simulink model "Nonlinear_Inverted_Pendulum_Modern"  (R2012b)
settings: Solver=ode45  StartTime=0.0  StopTime=STOP  FixedStep=T  RelTol=1e-3
values from neighbouring files (symbols this model uses):
  b = 0.1    [Nonlinear_Inverted_Pendulum_Modern_m.m]
  g = 9.8    [Nonlinear_Inverted_Pendulum_Modern_m.m]    (also in PolePlacement_m.m)
  I = 0.006    [Nonlinear_Inverted_Pendulum_Modern_m.m]    (also in PolePlacement_m.m)
  K = place(A,B,POLES)    [Nonlinear_Inverted_Pendulum_Modern_m.m]    (also in PolePlacement_m.m = -500)
  L = 0.3    [Nonlinear_Inverted_Pendulum_Modern_m.m]
  m = 0.2    [Nonlinear_Inverted_Pendulum_Modern_m.m]    (also in PolePlacement_m.m)
  M = 0.5    [Nonlinear_Inverted_Pendulum_Modern_m.m]    (also in PolePlacement_m.m)
  thetaInit = .1    (= 0.1)    [Nonlinear_Inverted_Pendulum_Modern_m.m]    (also in PolePlacement_m.m)
settings Model: Creator=Andrew  LastModifiedBy=Andrew
settings SolverCC: AlgebraicLoopSolver=LineSearch

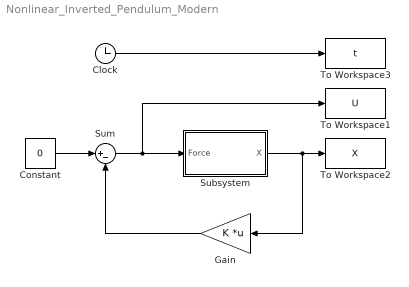
== system Nonlinear_Inverted_Pendulum_Modern ==
  Clock : Clock
  Constant : Constant  Value=0
  Gain : Gain  Gain=K  Multiplication=Matrix(K*u)
  Subsystem : Subsystem
  Sum : Sum  Inputs=|+-
  To Workspace1 : ToWorkspace  VariableName=U  SampleTime=-1
  To Workspace2 : ToWorkspace  VariableName=X  SampleTime=-1
  To Workspace3 : ToWorkspace  VariableName=t  SampleTime=-1
  wires:
  Sum/1 -> Subsystem/1(Force), To Workspace1/1
  Subsystem/1(X) -> To Workspace2/1, Gain/1
  Constant/1 -> Sum/1
  Clock/1 -> To Workspace3/1
  Gain/1 -> Sum/2

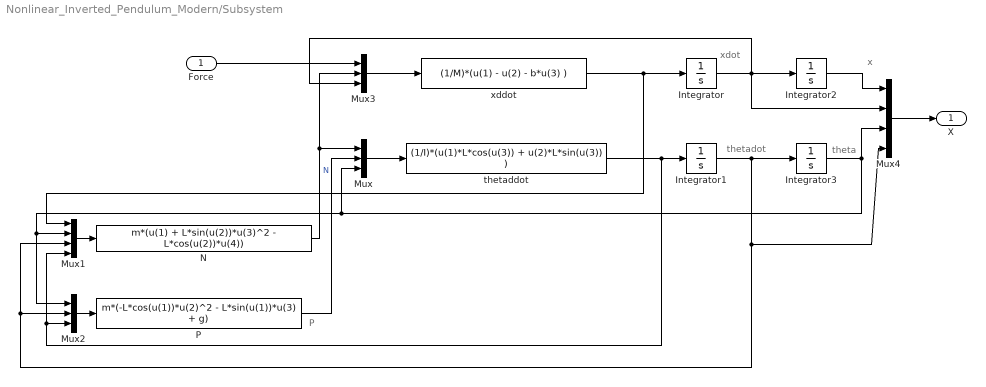
== system Nonlinear_Inverted_Pendulum_Modern/Subsystem ==
  note: xdot
  note: x
  note: thetadot
  note: theta
  note: P
  Force : Inport
  Integrator : Integrator  ContinuousStateAttributes='xdot'
  Integrator1 : Integrator  ContinuousStateAttributes='thetadot'
  Integrator2 : Integrator  ContinuousStateAttributes='x'
  Integrator3 : Integrator  InitialCondition=thetaInit  ContinuousStateAttributes='theta'
  Mux : Mux  Inputs=3
  Mux1 : Mux
  Mux2 : Mux  Inputs=3
  Mux3 : Mux  Inputs=3
  Mux4 : Mux
  N : Fcn  Expr=m*(u(1) + L*sin(u(2))*u(3)^2 - L*cos(u(2))*u(4))
  P : Fcn  Expr=m*(-L*cos(u(1))*u(2)^2 - L*sin(u(1))*u(3) + g)
  thetaddot : Fcn  Expr=(1/I)*(u(1)*L*cos(u(3)) + u(2)*L*sin(u(3)) )
  xddot : Fcn  Expr=(1/M)*(u(1) - u(2) - b*u(3) )
  X : Outport
  wires:
  Integrator/1 -> Mux4/2, Integrator2/1, Mux3/3
  Integrator1/1 -> Mux4/4, Mux1/3, Mux2/2, Integrator3/1
  xddot/1 -> Integrator/1, Mux1/1
  thetaddot/1 -> Mux1/4, Mux2/3, Integrator1/1
  Mux/1 -> thetaddot/1
  Integrator3/1 -> Mux4/3, Mux2/1, Mux1/2, Mux/3
  Mux1/1 -> N/1
  Mux3/1 -> xddot/1
  Force/1 -> Mux3/1
  N/1 -> Mux/1, Mux3/2  "N"
  Mux2/1 -> P/1
  P/1 -> Mux/2
  Integrator2/1 -> Mux4/1
  Mux4/1 -> X/1
